simulink model "ctrl_DP_basic"  (R2015a)
settings: Solver=ode4  StartTime=0.0  StopTime=inf  FixedStep=0.01  RelTol=1e-3
values from neighbouring files (symbols this model uses):
  C = [C1;C2;C3;C4;C5;C6]    [initfile.m]    (also in thrustallocationQuadraticFixed.m)
  D = 3.0/100    (= 0.03)    [initfile.m]    (also in thrustallocationQuadraticFixed.m = 0.0411111111111)
  eps_c = 5    [initfile.m]
  epsilon = 0.5    [initfile.m]    (also in thrustallocationPseudo.m = u(10); thrustallocationQuadraticFixed.m = u(10))
  hd = c2d(H1,0.01,'foh')    [initfile.m]
  hd2 = c2d(H2,0.01,'zoh')    [initfile.m]
  I_s = 25000 /747225    (= 0.0334571246947)    [initfile.m]
  k_cc = 1    [initfile.m]
  K_omega = 0.3    [initfile.m]
  Kp = 3.3    [initfile.m]
  Max_Acceleration = 5    [initfile.m]
  Max_rotation = 12*sqrt(lambda)    [initfile.m]
  Max_thrust = 1.5    [initfile.m]
  n_c = 5    [initfile.m]
  p_cc = 0.5    [initfile.m]
  Q_f0 = 0.3    [initfile.m]
  r_cc = 4    [initfile.m]
  Rho = Rho_m    (= 1000)    [initfile.m]
undefined symbols (not defined in the file or in its folder): Kq, Kqr, Kt, Ktr, n_max, P_max, Q_max, shaft_to_pwm_coeff, thrust_to_pwm_coeff, Thruster, Thruster_control, Thruster_lock
libraries: marine_gnc x9, simulink x6, simulink_extras x2
(part 2 of 5)

== system ctrl_DP_basic/Guidance output ==
  Demux1 : Demux  Outputs=3
  Demux2 : Demux  Outputs=3
  Transposed rotation matrix in yaw2 : marine_gnc/Models/ Kinematics/Transposed rotation  matrix in yaw
  eta1 : ToFile  Commented=on  Filename=eta_d.mat  MatrixName=eta_d
  eta2 : ToFile  Commented=on  Filename=ref.mat  MatrixName=ref
  nu 1 : ToFile  Commented=on  Filename=eta_dot_d.mat  MatrixName=eta_dot_d
  nu_dot1 : ToFile  Commented=on  Filename=eta_ddot_d.mat  MatrixName=eta_ddot_d
  psi_d : S-Function  Priority=3  FunctionName=NIVeriStandIO  Parameters=width dtype portnum stime stype btype  mask(NI VeriStand Outport){portnum=3, width=-1, stime=-1, dtype=auto, stype=auto, btype=0}
      mask prompts: portnum "Port number:"; width "Port dimensions (-1 for dynamically sized):"; stime "Sample time (-1 for inherited):"; dtype "Data type:"; stype "Signal type:"; btype "Block type:"
      mask help: Use this outport on any level of nested subsystems to allow NI VeriStand software to map signals to it.
      mask init:
      | NIVeriStandIO_init;
      settings: CopyFcn=NIVeriStand_MDL_functions('', 'IO_copy');  DeleteFcn=NIVeriStand_MDL_functions('', 'IO_delete');  MoveFcn=set_param(gcb, 'Mask', 'on');
      mask Callback portnum: NIVeriStand_MDL_functions('', 'IO_setportnum');
      mask TypeOptions dtype: auto | double | single | int8 | uint8 | int16 | uint16 | int32 | uint32 | boolean
      mask Callback dtype: NIVeriStand_MDL_functions('', 'IO_booleansignal');
      mask TypeOptions stype: auto | real | complex
      mask Display:
      | patch([-x x], [-y y], [.90980 .81960 .32156]);
      | plot([xrad -x x xrad], [yrad -y y yrad]);
      | fprintf('NI Out%d', portnum);
  r_d : S-Function  Priority=4  FunctionName=NIVeriStandIO  Parameters=width dtype portnum stime stype btype  mask(NI VeriStand Outport){portnum=4, width=-1, stime=-1, dtype=auto, stype=auto, btype=0}
      mask prompts: portnum "Port number:"; width "Port dimensions (-1 for dynamically sized):"; stime "Sample time (-1 for inherited):"; dtype "Data type:"; stype "Signal type:"; btype "Block type:"
      mask help: Use this outport on any level of nested subsystems to allow NI VeriStand software to map signals to it.
      mask init:
      | NIVeriStandIO_init;
      settings: CopyFcn=NIVeriStand_MDL_functions('', 'IO_copy');  DeleteFcn=NIVeriStand_MDL_functions('', 'IO_delete');  MoveFcn=set_param(gcb, 'Mask', 'on');
      mask Callback portnum: NIVeriStand_MDL_functions('', 'IO_setportnum');
      mask TypeOptions dtype: auto | double | single | int8 | uint8 | int16 | uint16 | int32 | uint32 | boolean
      mask Callback dtype: NIVeriStand_MDL_functions('', 'IO_booleansignal');
      mask TypeOptions stype: auto | real | complex
      mask Display:
      | patch([-x x], [-y y], [.90980 .81960 .32156]);
      | plot([xrad -x x xrad], [yrad -y y yrad]);
      | fprintf('NI Out%d', portnum);
  u_d : S-Function  Priority=5  FunctionName=NIVeriStandIO  Parameters=width dtype portnum stime stype btype  mask(NI VeriStand Outport){portnum=5, width=-1, stime=-1, dtype=auto, stype=auto, btype=0}
      mask prompts: portnum "Port number:"; width "Port dimensions (-1 for dynamically sized):"; stime "Sample time (-1 for inherited):"; dtype "Data type:"; stype "Signal type:"; btype "Block type:"
      mask help: Use this outport on any level of nested subsystems to allow NI VeriStand software to map signals to it.
      mask init:
      | NIVeriStandIO_init;
      settings: CopyFcn=NIVeriStand_MDL_functions('', 'IO_copy');  DeleteFcn=NIVeriStand_MDL_functions('', 'IO_delete');  MoveFcn=set_param(gcb, 'Mask', 'on');
      mask Callback portnum: NIVeriStand_MDL_functions('', 'IO_setportnum');
      mask TypeOptions dtype: auto | double | single | int8 | uint8 | int16 | uint16 | int32 | uint32 | boolean
      mask Callback dtype: NIVeriStand_MDL_functions('', 'IO_booleansignal');
      mask TypeOptions stype: auto | real | complex
      mask Display:
      | patch([-x x], [-y y], [.90980 .81960 .32156]);
      | plot([xrad -x x xrad], [yrad -y y yrad]);
      | fprintf('NI Out%d', portnum);
  v_d : S-Function  Priority=6  FunctionName=NIVeriStandIO  Parameters=width dtype portnum stime stype btype  mask(NI VeriStand Outport){portnum=6, width=-1, stime=-1, dtype=auto, stype=auto, btype=0}
      mask prompts: portnum "Port number:"; width "Port dimensions (-1 for dynamically sized):"; stime "Sample time (-1 for inherited):"; dtype "Data type:"; stype "Signal type:"; btype "Block type:"
      mask help: Use this outport on any level of nested subsystems to allow NI VeriStand software to map signals to it.
      mask init:
      | NIVeriStandIO_init;
      settings: CopyFcn=NIVeriStand_MDL_functions('', 'IO_copy');  DeleteFcn=NIVeriStand_MDL_functions('', 'IO_delete');  MoveFcn=set_param(gcb, 'Mask', 'on');
      mask Callback portnum: NIVeriStand_MDL_functions('', 'IO_setportnum');
      mask TypeOptions dtype: auto | double | single | int8 | uint8 | int16 | uint16 | int32 | uint32 | boolean
      mask Callback dtype: NIVeriStand_MDL_functions('', 'IO_booleansignal');
      mask TypeOptions stype: auto | real | complex
      mask Display:
      | patch([-x x], [-y y], [.90980 .81960 .32156]);
      | plot([xrad -x x xrad], [yrad -y y yrad]);
      | fprintf('NI Out%d', portnum);
  x_d : S-Function  Priority=1  FunctionName=NIVeriStandIO  Parameters=width dtype portnum stime stype btype  mask(NI VeriStand Outport){portnum=1, width=-1, stime=-1, dtype=auto, stype=auto, btype=0}
      mask prompts: portnum "Port number:"; width "Port dimensions (-1 for dynamically sized):"; stime "Sample time (-1 for inherited):"; dtype "Data type:"; stype "Signal type:"; btype "Block type:"
      mask help: Use this outport on any level of nested subsystems to allow NI VeriStand software to map signals to it.
      mask init:
      | NIVeriStandIO_init;
      settings: CopyFcn=NIVeriStand_MDL_functions('', 'IO_copy');  DeleteFcn=NIVeriStand_MDL_functions('', 'IO_delete');  MoveFcn=set_param(gcb, 'Mask', 'on');
      mask Callback portnum: NIVeriStand_MDL_functions('', 'IO_setportnum');
      mask TypeOptions dtype: auto | double | single | int8 | uint8 | int16 | uint16 | int32 | uint32 | boolean
      mask Callback dtype: NIVeriStand_MDL_functions('', 'IO_booleansignal');
      mask TypeOptions stype: auto | real | complex
      mask Display:
      | patch([-x x], [-y y], [.90980 .81960 .32156]);
      | plot([xrad -x x xrad], [yrad -y y yrad]);
      | fprintf('NI Out%d', portnum);
  y_d : S-Function  Priority=2  FunctionName=NIVeriStandIO  Parameters=width dtype portnum stime stype btype  mask(NI VeriStand Outport){portnum=2, width=-1, stime=-1, dtype=auto, stype=auto, btype=0}
      mask prompts: portnum "Port number:"; width "Port dimensions (-1 for dynamically sized):"; stime "Sample time (-1 for inherited):"; dtype "Data type:"; stype "Signal type:"; btype "Block type:"
      mask help: Use this outport on any level of nested subsystems to allow NI VeriStand software to map signals to it.
      mask init:
      | NIVeriStandIO_init;
      settings: CopyFcn=NIVeriStand_MDL_functions('', 'IO_copy');  DeleteFcn=NIVeriStand_MDL_functions('', 'IO_delete');  MoveFcn=set_param(gcb, 'Mask', 'on');
      mask Callback portnum: NIVeriStand_MDL_functions('', 'IO_setportnum');
      mask TypeOptions dtype: auto | double | single | int8 | uint8 | int16 | uint16 | int32 | uint32 | boolean
      mask Callback dtype: NIVeriStand_MDL_functions('', 'IO_booleansignal');
      mask TypeOptions stype: auto | real | complex
      mask Display:
      | patch([-x x], [-y y], [.90980 .81960 .32156]);
      | plot([xrad -x x xrad], [yrad -y y yrad]);
      | fprintf('NI Out%d', portnum);
  wires:
  [eta_d] -> Demux1/1, eta1/1
  [eta_ddot_d] -> nu_dot1/1
  [ref] -> eta2/1
  Demux1/1 -> x_d/1
  Demux1/2 -> y_d/1
  Demux1/3 -> Transposed rotation matrix in yaw2/1, psi_d/1
  [eta_dot_d] -> nu 1/1, Transposed rotation matrix in yaw2/2
  Demux2/1 -> u_d/1
  Demux2/2 -> v_d/1
  Demux2/3 -> r_d/1
  Transposed rotation matrix in yaw2/1 -> Demux2/1

== system ctrl_DP_basic/Input ==
  Control Gains : Subsystem
  Guidance gains : Subsystem
  Mux : Mux  Inputs=3
  Observer Gains : Subsystem
  psi_ref : S-Function  Priority=2  FunctionName=NIVeriStandIO  Parameters=width dtype portnum stime stype btype  mask(NI VeriStand Inport){portnum=2, width=-1, stime=-1, dtype=auto, stype=auto, btype=1}
      mask prompts: portnum "Port number:"; width "Port dimensions (-1 for dynamically sized):"; stime "Sample time (-1 for inherited):"; dtype "Data type:"; stype "Signal type:"; btype "Block type:"
      mask help: Use this inport on any level of nested subsystems to allow NI VeriStand software to map signals to it.
      mask init:
      | NIVeriStandIO_init;
      settings: CopyFcn=NIVeriStand_MDL_functions('', 'IO_copy');  DeleteFcn=NIVeriStand_MDL_functions('', 'IO_delete');  MoveFcn=set_param(gcb, 'Mask', 'on');
      mask Callback portnum: NIVeriStand_MDL_functions('', 'IO_setportnum');
      mask TypeOptions dtype: auto | double | single | int8 | uint8 | int16 | uint16 | int32 | uint32 | boolean
      mask Callback dtype: NIVeriStand_MDL_functions('', 'IO_booleansignal');
      mask TypeOptions stype: auto | real | complex
      mask Display:
      | patch([-x x], [-y y], [.90980 .81960 .32156]);
      | plot([xrad -x x xrad], [yrad -y y yrad]);
      | fprintf('NI In%d', portnum);
  reset : S-Function  Priority=1  FunctionName=NIVeriStandIO  Parameters=width dtype portnum stime stype btype  mask(NI VeriStand Inport){portnum=1, width=-1, stime=-1, dtype=auto, stype=auto, btype=1}
      mask prompts: portnum "Port number:"; width "Port dimensions (-1 for dynamically sized):"; stime "Sample time (-1 for inherited):"; dtype "Data type:"; stype "Signal type:"; btype "Block type:"
      mask help: Use this inport on any level of nested subsystems to allow NI VeriStand software to map signals to it.
      mask init:
      | NIVeriStandIO_init;
      settings: CopyFcn=NIVeriStand_MDL_functions('', 'IO_copy');  DeleteFcn=NIVeriStand_MDL_functions('', 'IO_delete');  MoveFcn=set_param(gcb, 'Mask', 'on');
      mask Callback portnum: NIVeriStand_MDL_functions('', 'IO_setportnum');
      mask TypeOptions dtype: auto | double | single | int8 | uint8 | int16 | uint16 | int32 | uint32 | boolean
      mask Callback dtype: NIVeriStand_MDL_functions('', 'IO_booleansignal');
      mask TypeOptions stype: auto | real | complex
      mask Display:
      | patch([-x x], [-y y], [.90980 .81960 .32156]);
      | plot([xrad -x x xrad], [yrad -y y yrad]);
      | fprintf('NI In%d', portnum);
  x_ref : S-Function  Priority=3  FunctionName=NIVeriStandIO  Parameters=width dtype portnum stime stype btype  mask(NI VeriStand Inport){portnum=3, width=-1, stime=-1, dtype=auto, stype=auto, btype=1}
      mask prompts: portnum "Port number:"; width "Port dimensions (-1 for dynamically sized):"; stime "Sample time (-1 for inherited):"; dtype "Data type:"; stype "Signal type:"; btype "Block type:"
      mask help: Use this inport on any level of nested subsystems to allow NI VeriStand software to map signals to it.
      mask init:
      | NIVeriStandIO_init;
      settings: CopyFcn=NIVeriStand_MDL_functions('', 'IO_copy');  DeleteFcn=NIVeriStand_MDL_functions('', 'IO_delete');  MoveFcn=set_param(gcb, 'Mask', 'on');
      mask Callback portnum: NIVeriStand_MDL_functions('', 'IO_setportnum');
      mask TypeOptions dtype: auto | double | single | int8 | uint8 | int16 | uint16 | int32 | uint32 | boolean
      mask Callback dtype: NIVeriStand_MDL_functions('', 'IO_booleansignal');
      mask TypeOptions stype: auto | real | complex
      mask Display:
      | patch([-x x], [-y y], [.90980 .81960 .32156]);
      | plot([xrad -x x xrad], [yrad -y y yrad]);
      | fprintf('NI In%d', portnum);
  y_ref : S-Function  Priority=4  FunctionName=NIVeriStandIO  Parameters=width dtype portnum stime stype btype  mask(NI VeriStand Inport){portnum=4, width=-1, stime=-1, dtype=auto, stype=auto, btype=1}
      mask prompts: portnum "Port number:"; width "Port dimensions (-1 for dynamically sized):"; stime "Sample time (-1 for inherited):"; dtype "Data type:"; stype "Signal type:"; btype "Block type:"
      mask help: Use this inport on any level of nested subsystems to allow NI VeriStand software to map signals to it.
      mask init:
      | NIVeriStandIO_init;
      settings: CopyFcn=NIVeriStand_MDL_functions('', 'IO_copy');  DeleteFcn=NIVeriStand_MDL_functions('', 'IO_delete');  MoveFcn=set_param(gcb, 'Mask', 'on');
      mask Callback portnum: NIVeriStand_MDL_functions('', 'IO_setportnum');
      mask TypeOptions dtype: auto | double | single | int8 | uint8 | int16 | uint16 | int32 | uint32 | boolean
      mask Callback dtype: NIVeriStand_MDL_functions('', 'IO_booleansignal');
      mask TypeOptions stype: auto | real | complex
      mask Display:
      | patch([-x x], [-y y], [.90980 .81960 .32156]);
      | plot([xrad -x x xrad], [yrad -y y yrad]);
      | fprintf('NI In%d', portnum);
  reference : Outport
  tag scope: ref=global, reset=global
  wires:
  Mux/1 -> [ref], reference/1
  reset/1 -> [reset]
  x_ref/1 -> Mux/1
  y_ref/1 -> Mux/2
  psi_ref/1 -> Mux/3

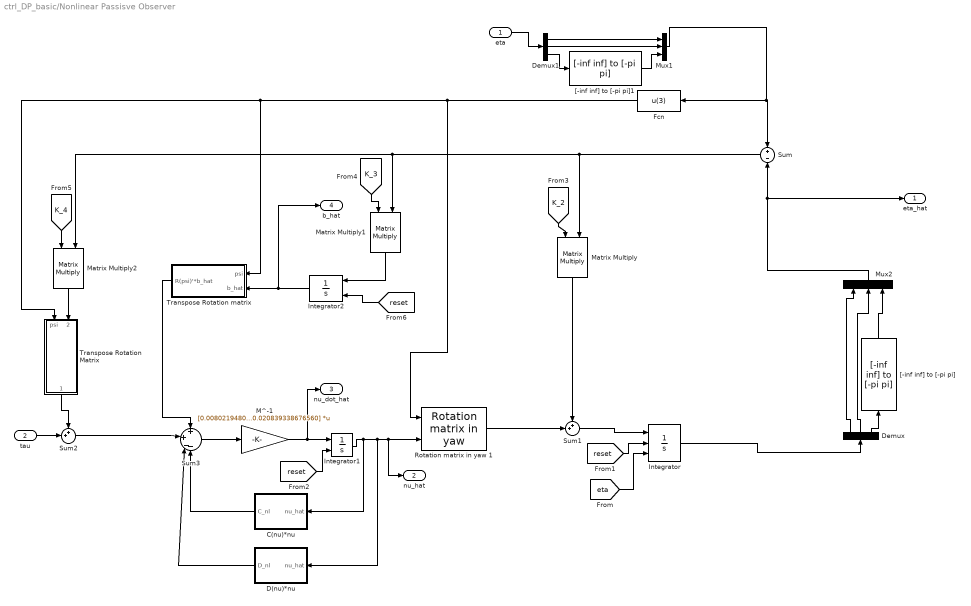
== system ctrl_DP_basic/Nonlinear Passisve Observer ==
  eta : Inport
  tau : Inport  Port=2
  C(nu)*nu : MATLAB Function  TreatAsAtomicUnit=on
  D(nu)*nu : MATLAB Function  TreatAsAtomicUnit=on
  Demux : Demux  Outputs=3
  Demux1 : Demux  Outputs=3
  Fcn : Fcn  Expr=u(3)
  Integrator : Integrator  ExternalReset=either  InitialConditionSource=external
  Integrator1 : Integrator  ExternalReset=either  InitialCondition=[0 0 0]'
  Integrator2 : Integrator  ExternalReset=either  InitialCondition=[0 0 0]'
  M^-1 : Gain  Gain=[0.008021948049864 0 0;0 0.010098125265799 1.104781662647098e-04;0 3.303823257820844e-05 0.020839338676560]  Multiplication=Matrix(K*u)
  Matrix Multiply : Product  Multiplication=Matrix(*)
  Matrix Multiply1 : Product  Multiplication=Matrix(*)
  Matrix Multiply2 : Product  Multiplication=Matrix(*)
  Mux1 : Mux  Inputs=3
  Mux2 : Mux  Inputs=3
  Rotation matrix in yaw 1 : marine_gnc/Models/ Kinematics/Rotation matrix in yaw 
  Sum : Sum  Inputs=+|-
  Sum1 : Sum  Inputs=++|
  Sum2 : Sum  Inputs=++|
  Sum3 : Sum  Inputs=+|+|--
  Transpose Rotation Matrix : Subsystem
  Transpose Rotation matrix : Subsystem
  "[-inf inf] to [-pi pi]" : marine_gnc/Utilities/Math Operations/[-inf inf] to [-pi pi]
  "[-inf inf] to [-pi pi]1" : marine_gnc/Utilities/Math Operations/[-inf inf] to [-pi pi]
  eta_hat : Outport
  nu_hat : Outport  Port=2
  nu_dot_hat : Outport  Port=3
  b_hat : Outport  Port=4
  wires:
  Mux1/1 -> Fcn/1, Sum/1
  Sum1/1 -> Integrator/1
  Mux2/1 -> Sum/2, eta_hat/1
  Matrix Multiply/1 -> Sum1/1
  Sum/1 -> Matrix Multiply2/2, Matrix Multiply1/2, Matrix Multiply/2
  Fcn/1 -> Rotation matrix in yaw 1/1, Transpose Rotation matrix/1(psi), Transpose Rotation Matrix/1(psi)
  tau/1 -> Sum2/2
  Matrix Multiply2/1 -> Transpose Rotation Matrix/2(y_tilde)
  Transpose Rotation Matrix/1(R(psi)'*y_tilde) -> Sum2/1
  Transpose Rotation matrix/1(R(psi)'*b_hat) -> Sum3/1
  Sum2/1 -> Sum3/2
  Sum3/1 -> M^-1/1
  M^-1/1 -> nu_dot_hat/1, Integrator1/1
  D(nu)*nu/1(D_nl) -> Sum3/3
  Integrator1/1 -> C(nu)*nu/1(nu_hat), Rotation matrix in yaw 1/2, nu_hat/1, D(nu)*nu/1(nu_hat)
  Rotation matrix in yaw 1/1 -> Sum1/2
  Integrator2/1 -> b_hat/1, Transpose Rotation matrix/2(b_hat)
  C(nu)*nu/1(C_nl) -> Sum3/4
  Demux/1 -> Mux2/1
  Demux/2 -> Mux2/2
  "[-inf inf] to [-pi pi]"/1 -> Mux2/3
  Demux/3 -> "[-inf inf] to [-pi pi]"/1
  Integrator/1 -> Demux/1
  Demux1/1 -> Mux1/1
  Demux1/2 -> Mux1/2
  "[-inf inf] to [-pi pi]1"/1 -> Mux1/3
  Demux1/3 -> "[-inf inf] to [-pi pi]1"/1
  eta/1 -> Demux1/1
  [eta] -> Integrator/3
  [reset] -> Integrator/2
  [reset] -> Integrator1/2
  [K_4] -> Matrix Multiply2/1
  [K_3] -> Matrix Multiply1/1
  [K_2] -> Matrix Multiply/1
  [reset] -> Integrator2/2
  Matrix Multiply1/1 -> Integrator2/1

== system ctrl_DP_basic/Observer output  ==
  eta_hat : Inport
  nu_hat : Inport  Port=2
  nu_dot_hat : Inport  Port=3
  b_hat : Inport  Port=4
  b_hat output : Subsystem
  eta_hat output : Subsystem
  nu_dot_hat output : Subsystem
  nu_hat output : Subsystem
  wires:
  eta_hat/1 -> eta_hat output/1(eta-_hat)
  nu_hat/1 -> nu_hat output/1(nu_hat)
  nu_dot_hat/1 -> nu_dot_hat output/1(nu_dot_hat)
  b_hat/1 -> b_hat output/1(b_hat)

== system ctrl_DP_basic/Parameters From initfile distributed  ==
  note: Propulsion Control
  Constant : Constant  Value=eps_c
  Constant1 : Constant  Value=k_cc
  Constant2 : Constant  Value=p_cc
  Constant3 : Constant  Value=r_cc
  Constant4 : Constant  Value=eps
  Constant5 : Constant  Value=n_c
  D : Constant  Value=D
  Kq : Constant  Value=Kq
  Kqr : Constant  Value=Kqr
  Kt : Constant  Value=Kt
  Ktr : Constant  Value=Ktr
  Rho : Constant  Value=Rho
  tag scope: D=global, Kq=global, Kqr=global, Kt=global, Ktr=global, Rho=global, eps=global, eps_c=global, k_cc=global, n_c=global, p_cc=global, r_cc=global
  wires:
  Kq/1 -> [Kq]
  Kt/1 -> [Kt]
  D/1 -> [D]
  Rho/1 -> [Rho]
  Constant/1 -> [eps_c]
  Constant1/1 -> [k_cc]
  Constant2/1 -> [p_cc]
  Constant3/1 -> [r_cc]
  Constant4/1 -> [eps]
  Kqr/1 -> [Kqr]
  Ktr/1 -> [Ktr]
  Constant5/1 -> [n_c]

== system ctrl_DP_basic/Thrust allocation1 ==
  tau : Inport
  Angles : Inport  Port=2
  "  Thrust calculated" : Selector  InputPortWidth=12  Indices=[7 8 9 10 11 12]
  " Angle calculated" : Selector  InputPortWidth=12  Indices=[1 2 3 4 5 6]
  C : Constant  Value=C
  Choosing Fixed / Azimuth angle : Switch  Threshold=1
  Constant to avoid singularities : Constant  Value=eps
  For Each Subsystem : Subsystem  TreatAsAtomicUnit=on
  MATLAB Function : MATLAB Function  TreatAsAtomicUnit=on
  Mux : Mux  Inputs=3
  Mux2 : Mux  Inputs=2
  Radians to Degrees : simulink_extras/Transformations/Radians to Degrees
  Switch Azimuth/Fixed angles : Constant  Value=Thruster_lock
  Thrust and angle specified : Selector  InputPortWidth=12  Indices=[7 1 8 2 9 3 10 4 11 5 12 6]
  X-position Thruster : Constant  Value=[Thruster.T1(1) Thruster.T2(1) Thruster.T3(1) Thruster.T4(1) Thruster.T5(1) Thruster.T6(1)]
  Y-position Thruster : Constant  Value=[Thruster.T1(2) Thruster.T2(2) Thruster.T3(2) Thruster.T4(2) Thruster.T5(2) Thruster.T6(2)]
  constant angle : Constant  Value=[Thruster.T1(3) Thruster.T2(3) Thruster.T3(3) Thruster.T4(3) Thruster.T5(3) Thruster.T6(3)]
  reset : S-Function  Priority=1  FunctionName=NIVeriStandIO  Parameters=width dtype portnum stime stype btype  mask(NI VeriStand Inport){portnum=1, width=-1, stime=-1, dtype=auto, stype=auto, btype=1}
      mask prompts: portnum "Port number:"; width "Port dimensions (-1 for dynamically sized):"; stime "Sample time (-1 for inherited):"; dtype "Data type:"; stype "Signal type:"; btype "Block type:"
      mask help: Use this inport on any level of nested subsystems to allow NI VeriStand software to map signals to it.
      mask init:
      | NIVeriStandIO_init;
      settings: CopyFcn=NIVeriStand_MDL_functions('', 'IO_copy');  DeleteFcn=NIVeriStand_MDL_functions('', 'IO_delete');  MoveFcn=set_param(gcb, 'Mask', 'on');
      mask Callback portnum: NIVeriStand_MDL_functions('', 'IO_setportnum');
      mask TypeOptions dtype: auto | double | single | int8 | uint8 | int16 | uint16 | int32 | uint32 | boolean
      mask Callback dtype: NIVeriStand_MDL_functions('', 'IO_booleansignal');
      mask TypeOptions stype: auto | real | complex
      mask Display:
      | patch([-x x], [-y y], [.90980 .81960 .32156]);
      | plot([xrad -x x xrad], [yrad -y y yrad]);
      | fprintf('NI In%d', portnum);
  Td & angle : Outport
  wires:
  Switch Azimuth/Fixed angles/1 -> Choosing Fixed / Azimuth angle/2
  Constant to avoid singularities/1 -> Mux/3
  " Angle calculated"/1 -> Choosing Fixed / Azimuth angle/1
  Thrust and angle specified/1 -> Td & angle/1
  Mux2/1 -> Thrust and angle specified/1
  "  Thrust calculated"/1 -> Mux2/2
  tau/1 -> Mux/1
  Choosing Fixed / Azimuth angle/1 -> For Each Subsystem/1(Desired Angle)
  Angles/1 -> Radians to Degrees/1
  For Each Subsystem/1("Out2 ") -> Mux2/1
  constant angle/1 -> For Each Subsystem/2("initial angle "), Choosing Fixed / Azimuth angle/3
  Radians to Degrees/1 -> Mux/2
  reset/1 -> For Each Subsystem/3(reset)
  MATLAB Function/1(sys) -> "  Thrust calculated"/1, " Angle calculated"/1
  Mux/1 -> MATLAB Function/1(u)
  X-position Thruster/1 -> MATLAB Function/2(ThrusterPosX)
  Y-position Thruster/1 -> MATLAB Function/3(ThrusterPosY)
  C/1 -> MATLAB Function/4(C)

== system ctrl_DP_basic/Thruster control  ==
  "Desired thrust and angle " : Inport
  Demux : Demux  Outputs=12
  Mux : Mux  Inputs=12
  Mux1 : Mux  Inputs=2
  Selecting Desired thrust1 : Selector  InputPortWidth=12  Indices=[1 3 5 7 9 11]
  Selecting actual angle : Selector  InputPortWidth=12  Indices=[2 4 6 8 10 12]
  Subsystem : Subsystem
  Subsystem1 : Subsystem
  Thruster 1 : Subsystem
      settings: AttributesFormatString=%<MinAlgLoopOccurrences>
  Thruster 2 : Subsystem
      settings: AttributesFormatString=%<MinAlgLoopOccurrences>
  Thruster 3 : Subsystem
      settings: AttributesFormatString=%<MinAlgLoopOccurrences>
  Thruster 4 : Subsystem
      settings: AttributesFormatString=%<MinAlgLoopOccurrences>
  Thruster 5 : Subsystem
      settings: AttributesFormatString=%<MinAlgLoopOccurrences>
  Thruster 6 : Subsystem
      settings: AttributesFormatString=%<MinAlgLoopOccurrences>
  "Commanded pwm " : Outport
  Commanded angle : Outport  Port=2
  Commanded thrust : Outport  Port=3
  wires:
  Selecting actual angle/1 -> Subsystem1/1(Calculated angles)
  "Desired thrust and angle "/1 -> Selecting actual angle/1, Selecting Desired thrust1/1
  Subsystem1/1(Commanded angles) -> Commanded angle/1
  Demux/1 -> Thruster 1/1(Desired thrust 1)
  Demux/2 -> Thruster 2/1(Desired thrust 1)
  Demux/3 -> Thruster 3/1(Desired thrust 1)
  Demux/4 -> Thruster 4/1(Desired thrust 1)
  Demux/5 -> Thruster 5/1(Desired thrust 1)
  Demux/6 -> Thruster 6/1(Desired thrust 1)
  Selecting Desired thrust1/1 -> Mux1/1
  Thruster 1/1("Commanded thrust ") -> Mux/1
  Thruster 1/2(Shaft speed) -> Mux/2
  Thruster 2/1("Commanded thrust ") -> Mux/3
  Thruster 3/1("Commanded thrust ") -> Mux/5
  Thruster 4/1("Commanded thrust ") -> Mux/7
  Thruster 5/1("Commanded thrust ") -> Mux/9
  Thruster 6/1("Commanded thrust ") -> Mux/11
  Thruster 2/2(Shaft speed) -> Mux/4
  Thruster 3/2(Shaft speed) -> Mux/6
  Thruster 4/2(Shaft speed) -> Mux/8
  Thruster 5/2(Shaft speed) -> Mux/10
  Thruster 6/2(Shaft speed) -> Mux/12
  Mux/1 -> Subsystem/1(Calculated thrust)
  Mux1/1 -> Demux/1
  Demux/7 -> Thruster 1/2(shaft speed)
  Demux/8 -> Thruster 2/2(shaft speed)
  Demux/9 -> Thruster 3/2(shaft speed)
  Demux/10 -> Thruster 4/2(shaft speed)
  Demux/11 -> Thruster 5/2(shaft speed)
  Demux/12 -> Thruster 6/2(shaft speed)
  Subsystem/1(pwm) -> "Commanded pwm "/1
  Subsystem/2(Force) -> Commanded thrust/1
  Subsystem/3(pwm to shaftspeed) -> Mux1/2

== system ctrl_DP_basic/Thruster measurment ==
  Mux1 : Mux  Inputs=6
  thr_angle_1 : S-Function  Priority=9  FunctionName=NIVeriStandIO  Parameters=width dtype portnum stime stype btype  mask(NI VeriStand Inport){portnum=9, width=-1, stime=-1, dtype=auto, stype=auto, btype=1}
      mask prompts: portnum "Port number:"; width "Port dimensions (-1 for dynamically sized):"; stime "Sample time (-1 for inherited):"; dtype "Data type:"; stype "Signal type:"; btype "Block type:"
      mask help: Use this inport on any level of nested subsystems to allow NI VeriStand software to map signals to it.
      mask init:
      | NIVeriStandIO_init;
      settings: CopyFcn=NIVeriStand_MDL_functions('', 'IO_copy');  DeleteFcn=NIVeriStand_MDL_functions('', 'IO_delete');  MoveFcn=set_param(gcb, 'Mask', 'on');
      mask Callback portnum: NIVeriStand_MDL_functions('', 'IO_setportnum');
      mask TypeOptions dtype: auto | double | single | int8 | uint8 | int16 | uint16 | int32 | uint32 | boolean
      mask Callback dtype: NIVeriStand_MDL_functions('', 'IO_booleansignal');
      mask TypeOptions stype: auto | real | complex
      mask Display:
      | patch([-x x], [-y y], [.90980 .81960 .32156]);
      | plot([xrad -x x xrad], [yrad -y y yrad]);
      | fprintf('NI In%d', portnum);
  thr_angle_2 : S-Function  Priority=4  FunctionName=NIVeriStandIO  Parameters=width dtype portnum stime stype btype  mask(NI VeriStand Inport){portnum=4, width=-1, stime=-1, dtype=auto, stype=auto, btype=1}
      mask prompts: portnum "Port number:"; width "Port dimensions (-1 for dynamically sized):"; stime "Sample time (-1 for inherited):"; dtype "Data type:"; stype "Signal type:"; btype "Block type:"
      mask help: Use this inport on any level of nested subsystems to allow NI VeriStand software to map signals to it.
      mask init:
      | NIVeriStandIO_init;
      settings: CopyFcn=NIVeriStand_MDL_functions('', 'IO_copy');  DeleteFcn=NIVeriStand_MDL_functions('', 'IO_delete');  MoveFcn=set_param(gcb, 'Mask', 'on');
      mask Callback portnum: NIVeriStand_MDL_functions('', 'IO_setportnum');
      mask TypeOptions dtype: auto | double | single | int8 | uint8 | int16 | uint16 | int32 | uint32 | boolean
      mask Callback dtype: NIVeriStand_MDL_functions('', 'IO_booleansignal');
      mask TypeOptions stype: auto | real | complex
      mask Display:
      | patch([-x x], [-y y], [.90980 .81960 .32156]);
      | plot([xrad -x x xrad], [yrad -y y yrad]);
      | fprintf('NI In%d', portnum);
  thr_angle_3 : S-Function  Priority=5  FunctionName=NIVeriStandIO  Parameters=width dtype portnum stime stype btype  mask(NI VeriStand Inport){portnum=5, width=-1, stime=-1, dtype=auto, stype=auto, btype=1}
      mask prompts: portnum "Port number:"; width "Port dimensions (-1 for dynamically sized):"; stime "Sample time (-1 for inherited):"; dtype "Data type:"; stype "Signal type:"; btype "Block type:"
      mask help: Use this inport on any level of nested subsystems to allow NI VeriStand software to map signals to it.
      mask init:
      | NIVeriStandIO_init;
      settings: CopyFcn=NIVeriStand_MDL_functions('', 'IO_copy');  DeleteFcn=NIVeriStand_MDL_functions('', 'IO_delete');  MoveFcn=set_param(gcb, 'Mask', 'on');
      mask Callback portnum: NIVeriStand_MDL_functions('', 'IO_setportnum');
      mask TypeOptions dtype: auto | double | single | int8 | uint8 | int16 | uint16 | int32 | uint32 | boolean
      mask Callback dtype: NIVeriStand_MDL_functions('', 'IO_booleansignal');
      mask TypeOptions stype: auto | real | complex
      mask Display:
      | patch([-x x], [-y y], [.90980 .81960 .32156]);
      | plot([xrad -x x xrad], [yrad -y y yrad]);
      | fprintf('NI In%d', portnum);
  thr_angle_4 : S-Function  Priority=6  FunctionName=NIVeriStandIO  Parameters=width dtype portnum stime stype btype  mask(NI VeriStand Inport){portnum=6, width=-1, stime=-1, dtype=auto, stype=auto, btype=1}
      mask prompts: portnum "Port number:"; width "Port dimensions (-1 for dynamically sized):"; stime "Sample time (-1 for inherited):"; dtype "Data type:"; stype "Signal type:"; btype "Block type:"
      mask help: Use this inport on any level of nested subsystems to allow NI VeriStand software to map signals to it.
      mask init:
      | NIVeriStandIO_init;
      settings: CopyFcn=NIVeriStand_MDL_functions('', 'IO_copy');  DeleteFcn=NIVeriStand_MDL_functions('', 'IO_delete');  MoveFcn=set_param(gcb, 'Mask', 'on');
      mask Callback portnum: NIVeriStand_MDL_functions('', 'IO_setportnum');
      mask TypeOptions dtype: auto | double | single | int8 | uint8 | int16 | uint16 | int32 | uint32 | boolean
      mask Callback dtype: NIVeriStand_MDL_functions('', 'IO_booleansignal');
      mask TypeOptions stype: auto | real | complex
      mask Display:
      | patch([-x x], [-y y], [.90980 .81960 .32156]);
      | plot([xrad -x x xrad], [yrad -y y yrad]);
      | fprintf('NI In%d', portnum);
  thr_angle_5 : S-Function  Priority=7  FunctionName=NIVeriStandIO  Parameters=width dtype portnum stime stype btype  mask(NI VeriStand Inport){portnum=7, width=-1, stime=-1, dtype=auto, stype=auto, btype=1}
      mask prompts: portnum "Port number:"; width "Port dimensions (-1 for dynamically sized):"; stime "Sample time (-1 for inherited):"; dtype "Data type:"; stype "Signal type:"; btype "Block type:"
      mask help: Use this inport on any level of nested subsystems to allow NI VeriStand software to map signals to it.
      mask init:
      | NIVeriStandIO_init;
      settings: CopyFcn=NIVeriStand_MDL_functions('', 'IO_copy');  DeleteFcn=NIVeriStand_MDL_functions('', 'IO_delete');  MoveFcn=set_param(gcb, 'Mask', 'on');
      mask Callback portnum: NIVeriStand_MDL_functions('', 'IO_setportnum');
      mask TypeOptions dtype: auto | double | single | int8 | uint8 | int16 | uint16 | int32 | uint32 | boolean
      mask Callback dtype: NIVeriStand_MDL_functions('', 'IO_booleansignal');
      mask TypeOptions stype: auto | real | complex
      mask Display:
      | patch([-x x], [-y y], [.90980 .81960 .32156]);
      | plot([xrad -x x xrad], [yrad -y y yrad]);
      | fprintf('NI In%d', portnum);
  thr_angle_6 : S-Function  Priority=8  FunctionName=NIVeriStandIO  Parameters=width dtype portnum stime stype btype  mask(NI VeriStand Inport){portnum=8, width=-1, stime=-1, dtype=auto, stype=auto, btype=1}
      mask prompts: portnum "Port number:"; width "Port dimensions (-1 for dynamically sized):"; stime "Sample time (-1 for inherited):"; dtype "Data type:"; stype "Signal type:"; btype "Block type:"
      mask help: Use this inport on any level of nested subsystems to allow NI VeriStand software to map signals to it.
      mask init:
      | NIVeriStandIO_init;
      settings: CopyFcn=NIVeriStand_MDL_functions('', 'IO_copy');  DeleteFcn=NIVeriStand_MDL_functions('', 'IO_delete');  MoveFcn=set_param(gcb, 'Mask', 'on');
      mask Callback portnum: NIVeriStand_MDL_functions('', 'IO_setportnum');
      mask TypeOptions dtype: auto | double | single | int8 | uint8 | int16 | uint16 | int32 | uint32 | boolean
      mask Callback dtype: NIVeriStand_MDL_functions('', 'IO_booleansignal');
      mask TypeOptions stype: auto | real | complex
      mask Display:
      | patch([-x x], [-y y], [.90980 .81960 .32156]);
      | plot([xrad -x x xrad], [yrad -y y yrad]);
      | fprintf('NI In%d', portnum);
  alpha_m : Outport
  wires:
  thr_angle_3/1 -> Mux1/3
  thr_angle_1/1 -> Mux1/1
  Mux1/1 -> alpha_m/1
  thr_angle_5/1 -> Mux1/5
  thr_angle_4/1 -> Mux1/4
  thr_angle_6/1 -> Mux1/6
  thr_angle_2/1 -> Mux1/2

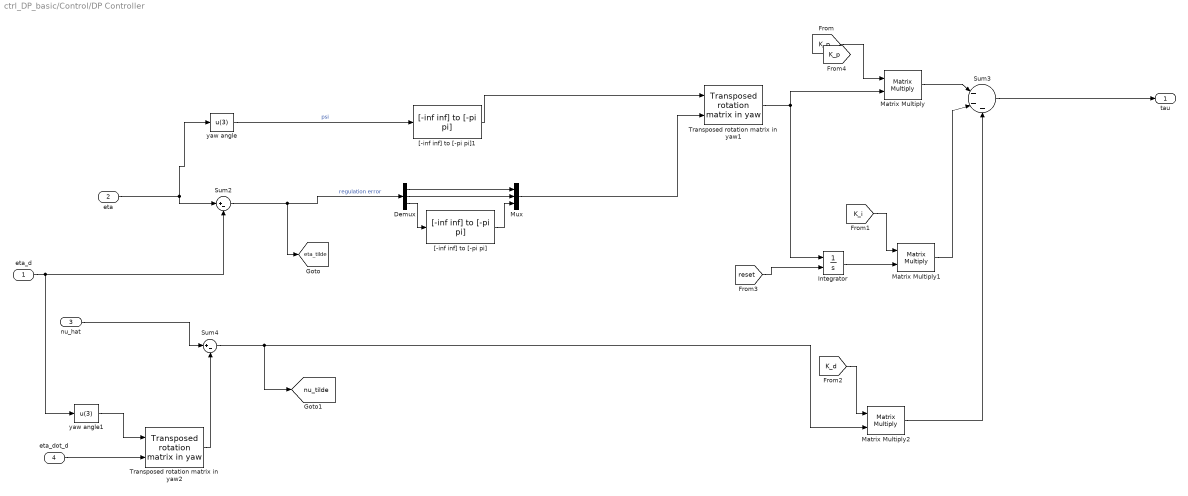
== system ctrl_DP_basic/Control/DP Controller ==
  eta_d : Inport
  eta : Inport  Port=2
  nu_hat : Inport  Port=3
  eta_dot_d : Inport  Port=4
  Demux : Demux  Outputs=3
  Integrator : Integrator  ExternalReset=either
  Matrix Multiply : Product  Multiplication=Matrix(*)
  Matrix Multiply1 : Product  Multiplication=Matrix(*)
  Matrix Multiply2 : Product  Multiplication=Matrix(*)
  Mux : Mux  Inputs=3
  Sum2 : Sum  Inputs=|+-  SaturateOnIntegerOverflow=on  InputSameDT=on  OutDataTypeStr=Inherit: Same as first input
  Sum3 : Sum  Inputs=|---  SaturateOnIntegerOverflow=on  InputSameDT=on  OutDataTypeStr=Inherit: Same as first input
  Sum4 : Sum  Inputs=|+-  SaturateOnIntegerOverflow=on  InputSameDT=on  OutDataTypeStr=Inherit: Same as first input
  Transposed rotation matrix in yaw1 : marine_gnc/Models/ Kinematics/Transposed rotation  matrix in yaw
  Transposed rotation matrix in yaw2 : marine_gnc/Models/ Kinematics/Transposed rotation  matrix in yaw
  "[-inf inf] to [-pi pi]" : marine_gnc/Utilities/Math Operations/[-inf inf] to [-pi pi]
  "[-inf inf] to [-pi pi]1" : marine_gnc/Utilities/Math Operations/[-inf inf] to [-pi pi]
  yaw angle : Fcn  Expr=u(3)
  yaw angle1 : Fcn  Expr=u(3)
  tau : Outport  InitialOutput=0
  tag scope: eta_tilde=global, nu_tilde=global
  wires:
  "[-inf inf] to [-pi pi]1"/1 -> Transposed rotation matrix in yaw1/1
  yaw angle/1 -> "[-inf inf] to [-pi pi]1"/1  "psi"
  Mux/1 -> Transposed rotation matrix in yaw1/2
  Demux/1 -> Mux/1
  Demux/2 -> Mux/2
  "[-inf inf] to [-pi pi]"/1 -> Mux/3
  Sum2/1 -> [eta_tilde], Demux/1  "regulation error"
  Demux/3 -> "[-inf inf] to [-pi pi]"/1
  eta/1 -> Sum2/1, yaw angle/1
  nu_hat/1 -> Sum4/1
  Matrix Multiply2/1 -> Sum3/3
  Integrator/1 -> Matrix Multiply1/2
  Matrix Multiply/1 -> Sum3/1
  Matrix Multiply1/1 -> Sum3/2
  Transposed rotation matrix in yaw1/1 -> Integrator/1, Matrix Multiply/2
  eta_d/1 -> yaw angle1/1, Sum2/2
  [reset] -> Integrator/2
  [K_p] -> Matrix Multiply/1
  [K_i] -> Matrix Multiply1/1
  [K_d] -> Matrix Multiply2/1
  eta_dot_d/1 -> Transposed rotation matrix in yaw2/2
  Transposed rotation matrix in yaw2/1 -> Sum4/2
  Sum4/1 -> [nu_tilde], Matrix Multiply2/2
  yaw angle1/1 -> Transposed rotation matrix in yaw2/1
  Sum3/1 -> tau/1

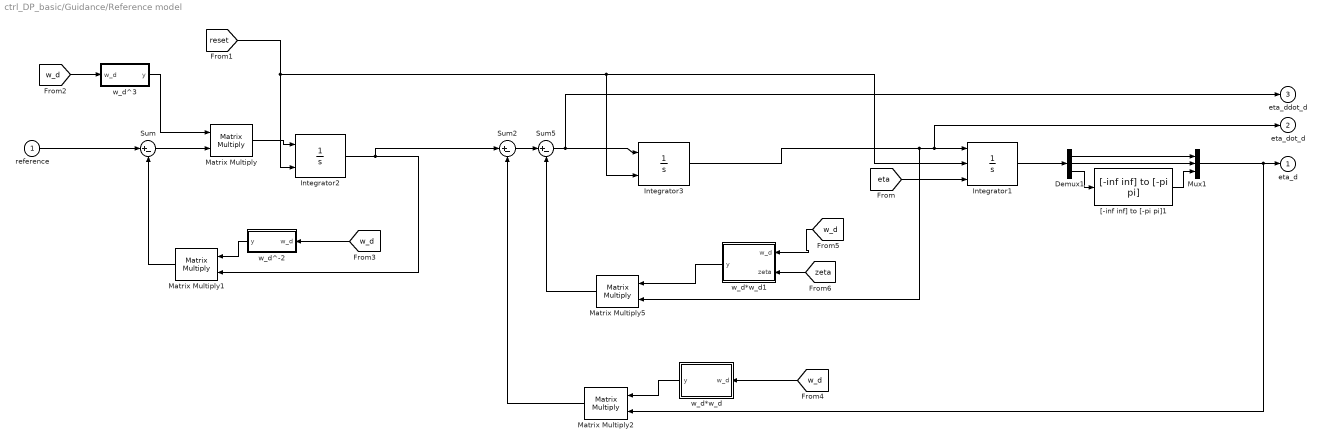
== system ctrl_DP_basic/Guidance/Reference model ==
  reference : Inport
  Demux1 : Demux  Outputs=3
  Integrator1 : Integrator  ExternalReset=either  InitialConditionSource=external
  Integrator2 : Integrator  ExternalReset=either
  Integrator3 : Integrator  ExternalReset=either
  Matrix Multiply{,1..2,5} (4 alike) : Product  Multiplication=Matrix(*)
  Mux1 : Mux  Inputs=3
  Sum : Sum  Inputs=|+-
  Sum2 : Sum  Inputs=|+-  SaturateOnIntegerOverflow=on  InputSameDT=on  OutDataTypeStr=Inherit: Same as first input
  Sum5 : Sum  Inputs=|+-  SaturateOnIntegerOverflow=on  InputSameDT=on  OutDataTypeStr=Inherit: Same as first input
  "[-inf inf] to [-pi pi]1" : marine_gnc/Utilities/Math Operations/[-inf inf] to [-pi pi]
  w_d*w_d : MATLAB Function  TreatAsAtomicUnit=on
  w_d*w_d1 : MATLAB Function  TreatAsAtomicUnit=on
  w_d^-2 : MATLAB Function  TreatAsAtomicUnit=on
  w_d^3 : MATLAB Function  TreatAsAtomicUnit=on
  eta_d : Outport  InitialOutput=0
  eta_dot_d : Outport  Port=2  InitialOutput=0
  eta_ddot_d : Outport  Port=3  InitialOutput=0
  wires:
  Integrator3/1 -> eta_dot_d/1, Integrator1/1, Matrix Multiply5/2
  Sum5/1 -> Integrator3/1, eta_ddot_d/1
  Integrator2/1 -> Sum2/1, Matrix Multiply1/2
  Sum2/1 -> Sum5/1
  Matrix Multiply2/1 -> Sum2/2
  Mux1/1 -> Matrix Multiply2/2, eta_d/1
  Matrix Multiply5/1 -> Sum5/2
  reference/1 -> Sum/1
  Sum/1 -> Matrix Multiply/2
  Matrix Multiply/1 -> Integrator2/1
  Matrix Multiply1/1 -> Sum/2
  [w_d] -> w_d^3/1(w_d)
  [w_d] -> w_d^-2/1(w_d)
  [w_d] -> w_d*w_d/1(w_d)
  w_d*w_d/1(y) -> Matrix Multiply2/1
  [zeta] -> w_d*w_d1/2(zeta)
  [w_d] -> w_d*w_d1/1(w_d)
  w_d*w_d1/1(y) -> Matrix Multiply5/1
  [eta] -> Integrator1/3
  [reset] -> Integrator3/2, Integrator1/2, Integrator2/2
  w_d^-2/1(y) -> Matrix Multiply1/1
  w_d^3/1(y) -> Matrix Multiply/1
  Demux1/1 -> Mux1/1
  "[-inf inf] to [-pi pi]1"/1 -> Mux1/3
  Demux1/3 -> "[-inf inf] to [-pi pi]1"/1
  Demux1/2 -> Mux1/2
  Integrator1/1 -> Demux1/1

== system ctrl_DP_basic/Input/Control Gains ==
  K_d_psi : S-Function  Priority=7  FunctionName=NIVeriStandIO  Parameters=width dtype portnum stime stype btype  mask(NI VeriStand Inport){portnum=7, width=-1, stime=-1, dtype=auto, stype=auto, btype=1}
      mask prompts: portnum "Port number:"; width "Port dimensions (-1 for dynamically sized):"; stime "Sample time (-1 for inherited):"; dtype "Data type:"; stype "Signal type:"; btype "Block type:"
      mask help: Use this inport on any level of nested subsystems to allow NI VeriStand software to map signals to it.
      mask init:
      | NIVeriStandIO_init;
      settings: CopyFcn=NIVeriStand_MDL_functions('', 'IO_copy');  DeleteFcn=NIVeriStand_MDL_functions('', 'IO_delete');  MoveFcn=set_param(gcb, 'Mask', 'on');
      mask Callback portnum: NIVeriStand_MDL_functions('', 'IO_setportnum');
      mask TypeOptions dtype: auto | double | single | int8 | uint8 | int16 | uint16 | int32 | uint32 | boolean
      mask Callback dtype: NIVeriStand_MDL_functions('', 'IO_booleansignal');
      mask TypeOptions stype: auto | real | complex
      mask Display:
      | patch([-x x], [-y y], [.90980 .81960 .32156]);
      | plot([xrad -x x xrad], [yrad -y y yrad]);
      | fprintf('NI In%d', portnum);
  K_d_x : S-Function  Priority=8  FunctionName=NIVeriStandIO  Parameters=width dtype portnum stime stype btype  mask(NI VeriStand Inport){portnum=8, width=-1, stime=-1, dtype=auto, stype=auto, btype=1}
      mask prompts: portnum "Port number:"; width "Port dimensions (-1 for dynamically sized):"; stime "Sample time (-1 for inherited):"; dtype "Data type:"; stype "Signal type:"; btype "Block type:"
      mask help: Use this inport on any level of nested subsystems to allow NI VeriStand software to map signals to it.
      mask init:
      | NIVeriStandIO_init;
      settings: CopyFcn=NIVeriStand_MDL_functions('', 'IO_copy');  DeleteFcn=NIVeriStand_MDL_functions('', 'IO_delete');  MoveFcn=set_param(gcb, 'Mask', 'on');
      mask Callback portnum: NIVeriStand_MDL_functions('', 'IO_setportnum');
      mask TypeOptions dtype: auto | double | single | int8 | uint8 | int16 | uint16 | int32 | uint32 | boolean
      mask Callback dtype: NIVeriStand_MDL_functions('', 'IO_booleansignal');
      mask TypeOptions stype: auto | real | complex
      mask Display:
      | patch([-x x], [-y y], [.90980 .81960 .32156]);
      | plot([xrad -x x xrad], [yrad -y y yrad]);
      | fprintf('NI In%d', portnum);
  K_d_y : S-Function  Priority=9  FunctionName=NIVeriStandIO  Parameters=width dtype portnum stime stype btype  mask(NI VeriStand Inport){portnum=9, width=-1, stime=-1, dtype=auto, stype=auto, btype=1}
      mask prompts: portnum "Port number:"; width "Port dimensions (-1 for dynamically sized):"; stime "Sample time (-1 for inherited):"; dtype "Data type:"; stype "Signal type:"; btype "Block type:"
      mask help: Use this inport on any level of nested subsystems to allow NI VeriStand software to map signals to it.
      mask init:
      | NIVeriStandIO_init;
      settings: CopyFcn=NIVeriStand_MDL_functions('', 'IO_copy');  DeleteFcn=NIVeriStand_MDL_functions('', 'IO_delete');  MoveFcn=set_param(gcb, 'Mask', 'on');
      mask Callback portnum: NIVeriStand_MDL_functions('', 'IO_setportnum');
      mask TypeOptions dtype: auto | double | single | int8 | uint8 | int16 | uint16 | int32 | uint32 | boolean
      mask Callback dtype: NIVeriStand_MDL_functions('', 'IO_booleansignal');
      mask TypeOptions stype: auto | real | complex
      mask Display:
      | patch([-x x], [-y y], [.90980 .81960 .32156]);
      | plot([xrad -x x xrad], [yrad -y y yrad]);
      | fprintf('NI In%d', portnum);
  K_i_psi : S-Function  Priority=4  FunctionName=NIVeriStandIO  Parameters=width dtype portnum stime stype btype  mask(NI VeriStand Inport){portnum=4, width=-1, stime=-1, dtype=auto, stype=auto, btype=1}
      mask prompts: portnum "Port number:"; width "Port dimensions (-1 for dynamically sized):"; stime "Sample time (-1 for inherited):"; dtype "Data type:"; stype "Signal type:"; btype "Block type:"
      mask help: Use this inport on any level of nested subsystems to allow NI VeriStand software to map signals to it.
      mask init:
      | NIVeriStandIO_init;
      settings: CopyFcn=NIVeriStand_MDL_functions('', 'IO_copy');  DeleteFcn=NIVeriStand_MDL_functions('', 'IO_delete');  MoveFcn=set_param(gcb, 'Mask', 'on');
      mask Callback portnum: NIVeriStand_MDL_functions('', 'IO_setportnum');
      mask TypeOptions dtype: auto | double | single | int8 | uint8 | int16 | uint16 | int32 | uint32 | boolean
      mask Callback dtype: NIVeriStand_MDL_functions('', 'IO_booleansignal');
      mask TypeOptions stype: auto | real | complex
      mask Display:
      | patch([-x x], [-y y], [.90980 .81960 .32156]);
      | plot([xrad -x x xrad], [yrad -y y yrad]);
      | fprintf('NI In%d', portnum);
  K_i_x : S-Function  Priority=5  FunctionName=NIVeriStandIO  Parameters=width dtype portnum stime stype btype  mask(NI VeriStand Inport){portnum=5, width=-1, stime=-1, dtype=auto, stype=auto, btype=1}
      mask prompts: portnum "Port number:"; width "Port dimensions (-1 for dynamically sized):"; stime "Sample time (-1 for inherited):"; dtype "Data type:"; stype "Signal type:"; btype "Block type:"
      mask help: Use this inport on any level of nested subsystems to allow NI VeriStand software to map signals to it.
      mask init:
      | NIVeriStandIO_init;
      settings: CopyFcn=NIVeriStand_MDL_functions('', 'IO_copy');  DeleteFcn=NIVeriStand_MDL_functions('', 'IO_delete');  MoveFcn=set_param(gcb, 'Mask', 'on');
      mask Callback portnum: NIVeriStand_MDL_functions('', 'IO_setportnum');
      mask TypeOptions dtype: auto | double | single | int8 | uint8 | int16 | uint16 | int32 | uint32 | boolean
      mask Callback dtype: NIVeriStand_MDL_functions('', 'IO_booleansignal');
      mask TypeOptions stype: auto | real | complex
      mask Display:
      | patch([-x x], [-y y], [.90980 .81960 .32156]);
      | plot([xrad -x x xrad], [yrad -y y yrad]);
      | fprintf('NI In%d', portnum);
  K_i_y : S-Function  Priority=6  FunctionName=NIVeriStandIO  Parameters=width dtype portnum stime stype btype  mask(NI VeriStand Inport){portnum=6, width=-1, stime=-1, dtype=auto, stype=auto, btype=1}
      mask prompts: portnum "Port number:"; width "Port dimensions (-1 for dynamically sized):"; stime "Sample time (-1 for inherited):"; dtype "Data type:"; stype "Signal type:"; btype "Block type:"
      mask help: Use this inport on any level of nested subsystems to allow NI VeriStand software to map signals to it.
      mask init:
      | NIVeriStandIO_init;
      settings: CopyFcn=NIVeriStand_MDL_functions('', 'IO_copy');  DeleteFcn=NIVeriStand_MDL_functions('', 'IO_delete');  MoveFcn=set_param(gcb, 'Mask', 'on');
      mask Callback portnum: NIVeriStand_MDL_functions('', 'IO_setportnum');
      mask TypeOptions dtype: auto | double | single | int8 | uint8 | int16 | uint16 | int32 | uint32 | boolean
      mask Callback dtype: NIVeriStand_MDL_functions('', 'IO_booleansignal');
      mask TypeOptions stype: auto | real | complex
      mask Display:
      | patch([-x x], [-y y], [.90980 .81960 .32156]);
      | plot([xrad -x x xrad], [yrad -y y yrad]);
      | fprintf('NI In%d', portnum);
  K_p_psi : S-Function  Priority=3  FunctionName=NIVeriStandIO  Parameters=width dtype portnum stime stype btype  mask(NI VeriStand Inport){portnum=3, width=-1, stime=-1, dtype=auto, stype=auto, btype=1}
      mask prompts: portnum "Port number:"; width "Port dimensions (-1 for dynamically sized):"; stime "Sample time (-1 for inherited):"; dtype "Data type:"; stype "Signal type:"; btype "Block type:"
      mask help: Use this inport on any level of nested subsystems to allow NI VeriStand software to map signals to it.
      mask init:
      | NIVeriStandIO_init;
      settings: CopyFcn=NIVeriStand_MDL_functions('', 'IO_copy');  DeleteFcn=NIVeriStand_MDL_functions('', 'IO_delete');  MoveFcn=set_param(gcb, 'Mask', 'on');
      mask Callback portnum: NIVeriStand_MDL_functions('', 'IO_setportnum');
      mask TypeOptions dtype: auto | double | single | int8 | uint8 | int16 | uint16 | int32 | uint32 | boolean
      mask Callback dtype: NIVeriStand_MDL_functions('', 'IO_booleansignal');
      mask TypeOptions stype: auto | real | complex
      mask Display:
      | patch([-x x], [-y y], [.90980 .81960 .32156]);
      | plot([xrad -x x xrad], [yrad -y y yrad]);
      | fprintf('NI In%d', portnum);
  K_p_x : S-Function  Priority=1  FunctionName=NIVeriStandIO  Parameters=width dtype portnum stime stype btype  mask(NI VeriStand Inport){portnum=1, width=-1, stime=-1, dtype=auto, stype=auto, btype=1}
      mask prompts: portnum "Port number:"; width "Port dimensions (-1 for dynamically sized):"; stime "Sample time (-1 for inherited):"; dtype "Data type:"; stype "Signal type:"; btype "Block type:"
      mask help: Use this inport on any level of nested subsystems to allow NI VeriStand software to map signals to it.
      mask init:
      | NIVeriStandIO_init;
      settings: CopyFcn=NIVeriStand_MDL_functions('', 'IO_copy');  DeleteFcn=NIVeriStand_MDL_functions('', 'IO_delete');  MoveFcn=set_param(gcb, 'Mask', 'on');
      mask Callback portnum: NIVeriStand_MDL_functions('', 'IO_setportnum');
      mask TypeOptions dtype: auto | double | single | int8 | uint8 | int16 | uint16 | int32 | uint32 | boolean
      mask Callback dtype: NIVeriStand_MDL_functions('', 'IO_booleansignal');
      mask TypeOptions stype: auto | real | complex
      mask Display:
      | patch([-x x], [-y y], [.90980 .81960 .32156]);
      | plot([xrad -x x xrad], [yrad -y y yrad]);
      | fprintf('NI In%d', portnum);
  K_p_y : S-Function  Priority=2  FunctionName=NIVeriStandIO  Parameters=width dtype portnum stime stype btype  mask(NI VeriStand Inport){portnum=2, width=-1, stime=-1, dtype=auto, stype=auto, btype=1}
      mask prompts: portnum "Port number:"; width "Port dimensions (-1 for dynamically sized):"; stime "Sample time (-1 for inherited):"; dtype "Data type:"; stype "Signal type:"; btype "Block type:"
      mask help: Use this inport on any level of nested subsystems to allow NI VeriStand software to map signals to it.
      mask init:
      | NIVeriStandIO_init;
      settings: CopyFcn=NIVeriStand_MDL_functions('', 'IO_copy');  DeleteFcn=NIVeriStand_MDL_functions('', 'IO_delete');  MoveFcn=set_param(gcb, 'Mask', 'on');
      mask Callback portnum: NIVeriStand_MDL_functions('', 'IO_setportnum');
      mask TypeOptions dtype: auto | double | single | int8 | uint8 | int16 | uint16 | int32 | uint32 | boolean
      mask Callback dtype: NIVeriStand_MDL_functions('', 'IO_booleansignal');
      mask TypeOptions stype: auto | real | complex
      mask Display:
      | patch([-x x], [-y y], [.90980 .81960 .32156]);
      | plot([xrad -x x xrad], [yrad -y y yrad]);
      | fprintf('NI In%d', portnum);
  Kd : MATLAB Function  TreatAsAtomicUnit=on
  Ki : MATLAB Function  TreatAsAtomicUnit=on
  Kp : MATLAB Function  TreatAsAtomicUnit=on
  Mux1 : Mux  Inputs=3
  Mux2 : Mux  Inputs=3
  Mux3 : Mux  Inputs=3
  tag scope: K_d=global, K_i=global, K_p=global
  wires:
  K_p_x/1 -> Mux1/1
  K_p_psi/1 -> Mux1/3
  K_p_y/1 -> Mux1/2
  Mux1/1 -> Kp/1(K_p1)
  Kp/1(K_p) -> [K_p]
  Mux2/1 -> Ki/1(K_i1)
  K_d_x/1 -> Mux3/1
  K_d_psi/1 -> Mux3/3
  K_d_y/1 -> Mux3/2
  Mux3/1 -> Kd/1(K_d1)
  Ki/1(K_i) -> [K_i]
  Kd/1(K_d) -> [K_d]
  K_i_x/1 -> Mux2/1
  K_i_y/1 -> Mux2/2
  K_i_psi/1 -> Mux2/3
